simulink model "ques4"  (R2021a)
settings: Solver=VariableStepAuto  StartTime=0.0  StopTime=10.0  RelTol=1e-3
settings Model: Creator=AVM  LastModifiedBy=AVM

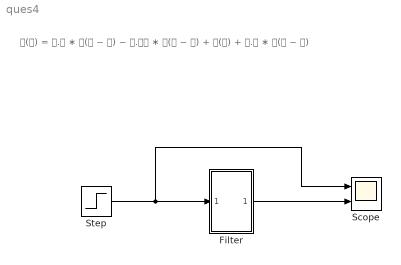
== system ques4 ==
  note: 𝐲(𝐧) = 𝟎.𝟓 ∗ 𝐲(𝐧 − 𝟏) − 𝟎.𝟐𝟓 ∗ 𝐲(𝐧 − 𝟐) + 𝐱(𝐧) + 𝟎.𝟒 ∗ 𝐱(𝐧 − 𝟏)
  Filter : Subsystem
  Scope : Scope  NumInputPorts=2
  Step : Step  SampleTime=0
  wires:
  Step/1 -> Scope/1, Filter/1(In1)
  Filter/1(Out1) -> Scope/2

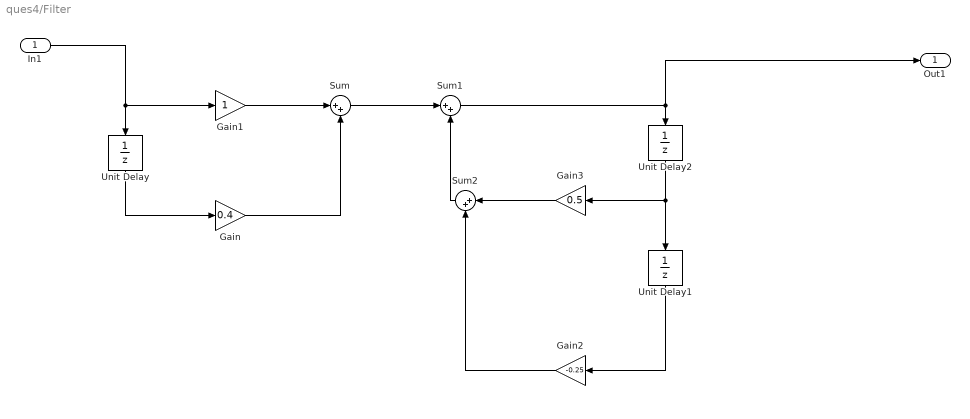
== system ques4/Filter ==
  In1 : Inport
  Gain : Gain  Gain=0.4
  Gain1 : Gain
  Gain2 : Gain  Gain=-0.25
  Gain3 : Gain  Gain=0.5
  Sum : Sum  Inputs=|++
  Sum1 : Sum  Inputs=|++
  Sum2 : Sum  Inputs=|++
  Unit Delay : UnitDelay  SampleTime=-1  HasFrameUpgradeWarning=on
  Unit Delay1 : UnitDelay  SampleTime=-1  HasFrameUpgradeWarning=on
  Unit Delay2 : UnitDelay  SampleTime=-1  HasFrameUpgradeWarning=on
  Out1 : Outport
  wires:
  Gain2/1 -> Sum2/2
  Unit Delay2/1 -> Gain3/1, Unit Delay1/1
  Gain1/1 -> Sum/1
  Sum1/1 -> Out1/1, Unit Delay2/1
  Unit Delay1/1 -> Gain2/1
  Unit Delay/1 -> Gain/1
  Sum2/1 -> Sum1/2
  Gain3/1 -> Sum2/1
  Gain/1 -> Sum/2
  Sum/1 -> Sum1/1
  In1/1 -> Unit Delay/1, Gain1/1
